simulink model "uplink_4c1r"  (Simulink 8.7)
settings: Solver=VariableStepDiscrete  StartTime=0.0  StopTime=DDC_Lineup_param.endTime  RelTol=1e-3
PreLoadFcn:
  | % Run the setup script when the model is opened
  | setup_uplink_4c1r;
InitFcn:
  | % Run the setup script again just before the
  | % model is run, so that any updates made
  | % after opening are applied.
  | setup_uplink_4c1r;
  | %% DSPBuilder Start
  | alt_dspbuilder_update_model(bdroot)
  | %% DSPBuilder End
undefined symbols (not defined in the file or in its folder): AdvDSPBChannelOutDisplay, carrier_separation, DDC_Lineup_param, dpoly, dspba_ChannelInVis, dspba_ChannelOutVis, dspba_internal_get_channel_ports, dspba_internal_get_demux_ports, evalAionMaskParam, latency, Power_Meter, primtype, Subsystem, uplink_4c1r_carrier_seperation_4c, uplink_4c1r_pd_accu_reg_block, uplink_4c1r_power_meter_1carrier, value
undefined symbols (not defined in the file): power_meter_param
libraries: DSPBAPrim x119, DSPBABase x26, uplink_4c1r_pipereg_lib x22, DSPBAModelBus x9, DSPBAFilters x5, uplink_4c1r_register x5, uplink_4c1r_accumulator x5, uplink_4c1r_peak_detector x5, uplink_4c1r_iq_square x4, DSPBAControl x2, DSPBAWaveformSynth x2, DSPBAUtilities x1
(part 2 of 3)

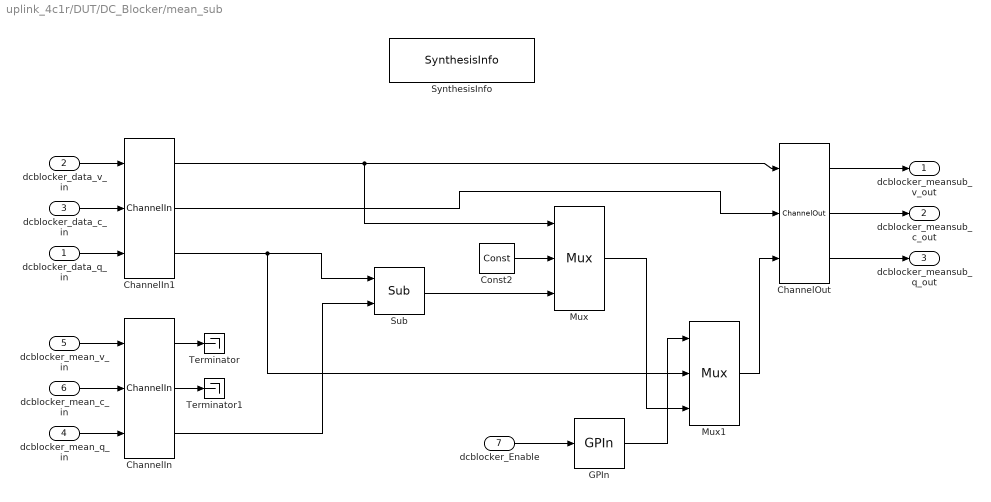
== system uplink_4c1r/DUT/DC_Blocker/mean_sub ==
  dcblocker_data_q_in : Inport
  dcblocker_data_v_in : Inport  Port=2
  dcblocker_data_c_in : Inport  Port=3
  dcblocker_mean_q_in : Inport  Port=4
  dcblocker_mean_v_in : Inport  Port=5
  dcblocker_mean_c_in : Inport  Port=6
  dcblocker_Enable : Inport  Port=7
  ChannelIn : DSPBAPrim/ChannelIn  primtype=channelin  nInputs=dspba_internal_get_channel_ports(gcb)  nOutputs=dspba_internal_get_channel_ports(gcb)  omode=Inherit via internal rule  otype=sfix(16)  scale=2^-15  rndmethod=Unbiased  factor=1  satmethod=Symmetric  shift_vec=[0 1 2 -1]  value=1  inPortNames=['v'; 'c'; '0'; '1'; '2'; '3'; '4'; '5'; '6'; '7'; '8'; '9'; 'A'; 'B'; 'D'; 'E'; 'F'; 'G'; 'H'; 'I'; 'J'; 'K'; 'L'; 'M'; 'N'; 'O'; 'P'; 'Q'; 'R'; 'S'; 'T'; 'U'; 'W'; 'X'; 'Y'; 'Z']  outPortNames=['v'; 'c'; '0'; '1'; '2'; '3'; '4'; '5'; '6'; '7'; '8'; '9'; 'A'; 'B'; 'D'; 'E'; 'F'; 'G'; 'H'; 'I'; 'J'; 'K'; 'L'; 'M'; 'N'; 'O'; 'P'; 'Q'; 'R'; 'S'; 'T'; 'U'; 'W'; 'X'; 'Y'; 'Z']  dspbaimage=dspba_prim.jpg  text=fprintf('In');  style=Optimised  dataSignals=1  foldingEnabled=off  channels=1  sampleRate=200  packetBeginPresent=off  packetBeginEnabled=off  visibilities=dspba_ChannelInVis(gcb)  latencyCorrection=0  version=20141013
  ChannelIn1 : DSPBAPrim/ChannelIn  primtype=channelin  nInputs=dspba_internal_get_channel_ports(gcb)  nOutputs=dspba_internal_get_channel_ports(gcb)  omode=Inherit via internal rule  otype=sfix(16)  scale=2^-15  rndmethod=Unbiased  factor=1  satmethod=Symmetric  shift_vec=[0 1 2 -1]  value=1  inPortNames=['v'; 'c'; '0'; '1'; '2'; '3'; '4'; '5'; '6'; '7'; '8'; '9'; 'A'; 'B'; 'D'; 'E'; 'F'; 'G'; 'H'; 'I'; 'J'; 'K'; 'L'; 'M'; 'N'; 'O'; 'P'; 'Q'; 'R'; 'S'; 'T'; 'U'; 'W'; 'X'; 'Y'; 'Z']  outPortNames=['v'; 'c'; '0'; '1'; '2'; '3'; '4'; '5'; '6'; '7'; '8'; '9'; 'A'; 'B'; 'D'; 'E'; 'F'; 'G'; 'H'; 'I'; 'J'; 'K'; 'L'; 'M'; 'N'; 'O'; 'P'; 'Q'; 'R'; 'S'; 'T'; 'U'; 'W'; 'X'; 'Y'; 'Z']  dspbaimage=dspba_prim.jpg  text=fprintf('In');  style=Optimised  dataSignals=1  foldingEnabled=off  channels=1  sampleRate=200  packetBeginPresent=off  packetBeginEnabled=off  visibilities=dspba_ChannelInVis(gcb)  latencyCorrection=0  version=20141013
  ChannelOut : DSPBAPrim/ChannelOut  primtype=channelout  nInputs=dspba_internal_get_channel_ports(gcb)  nOutputs=dspba_internal_get_channel_ports(gcb)  omode=Inherit via internal rule  otype=sfix(16)  scale=2^-15  rndmethod=Unbiased  factor=1  satmethod=Symmetric  shift_vec=[0 1 2 -1]  value=1  inPortNames=['v'; 'c'; '0'; '1'; '2'; '3'; '4'; '5'; '6'; '7'; '8'; '9'; 'A'; 'B'; 'D'; 'E'; 'F'; 'G'; 'H'; 'I'; 'J'; 'K'; 'L'; 'M'; 'N'; 'O'; 'P'; 'Q'; 'R'; 'S'; 'T'; 'U'; 'W'; 'X'; 'Y'; 'Z']  outPortNames=['v'; 'c'; '0'; '1'; '2'; '3'; '4'; '5'; '6'; '7'; '8'; '9'; 'A'; 'B'; 'D'; 'E'; 'F'; 'G'; 'H'; 'I'; 'J'; 'K'; 'L'; 'M'; 'N'; 'O'; 'P'; 'Q'; 'R'; 'S'; 'T'; 'U'; 'W'; 'X'; 'Y'; 'Z']  dspbaimage=dspba_prim.jpg  text=fprintf('Out%s', AdvDSPBChannelOutDisplay(latency));  style=Optimised  dataSignals=1  foldingEnabled=off  channels=1  sampleRate=200  packetBeginPresent=off  packetBeginEnabled=off  visibilities=dspba_ChannelOutVis(gcb)  latency=21  latencyCorrection=0  version=20141013
  Const2 : DSPBAPrim/Const  primtype=const  nInputs=0  nOutputs=1  omode=Specify via dialog  otype=sfix(16)  scale=2^-15  rndmethod=Unbiased  factor=1  satmethod=Symmetric  shift_vec=[0 1 2 -1]  value=0  inPortNames=['+'; '+';]  outPortNames=[' ']  dspbaimage=dspba_prim.jpg  text=fprintf('%s', num2str(value));  style=Optimised  visibilities=8 + 1024  floatPrecision=float32_m23  version=20120820
  GPIn : DSPBAPrim/GPIn  primtype=gpin  nInputs=evalAionMaskParam(gcb,'value',1)  nOutputs=evalAionMaskParam(gcb,'value',1)  omode=Inherit via internal rule  otype=sfix(16)  scale=2^-15  rndmethod=Unbiased  factor=1  satmethod=Symmetric  shift_vec=[0 1 2 -1]  value=1  inPortNames=[' ' ' ' ' ' ' ' ' ' ' ' ' ' ' ' ' ' ' ' ' ' ' ' ' ' ' ' ' ' ' ' ' ' ' ' ' ' ' ' ' ' ' ' ' ' ' ' ' ' ' ' ' ' ' ' ' ' ' ' ' ' ' ' ' ' ' ' ' ']'  outPortNames=[' ' ' ' ' ' ' ' ' ' ' ' ' ' ' ' ' ' ' ' ' ' ' ' ' ' ' ' ' ' ' ' ' ' ' ' ' ' ' ' ' ' ' ' ' ' ' ' ' ' ' ' ' ' ' ' ' ' ' ' ' ' ' ' ' ' ' ' ' ']'  dspbaimage=dspba_prim.jpg  text=fprintf('GPIn');  style=Optimised  visibilities=1024  latencyCorrection=0  version=20090407
  Mux : DSPBAPrim/Mux  primtype=mux  nInputs=evalAionMaskParam(gcb,'value',1)+1  nOutputs=1  omode=Inherit via internal rule  otype=sfix(16)  scale=2^-15  rndmethod=Unbiased  factor=1  satmethod=Symmetric  shift_vec=[0 1 2 -1]  value=2  inPortNames=['s'; 'd0'; 'd1'; 'd2'; 'd3'; 'd4'; 'd5'; 'd6'; 'd7'; 'd8'; 'd9';]  outPortNames=[' ']  dspbaimage=dspba_prim.jpg  text=fprintf('%s', primtype);  style=Optimised  visibilities=1032  version=20131025
  Mux1 : DSPBAPrim/Mux  primtype=mux  nInputs=evalAionMaskParam(gcb,'value',1)+1  nOutputs=1  omode=Inherit via internal rule  otype=sfix(16)  scale=2^-15  rndmethod=Unbiased  factor=1  satmethod=Symmetric  shift_vec=[0 1 2 -1]  value=2  inPortNames=['s'; 'd0'; 'd1'; 'd2'; 'd3'; 'd4'; 'd5'; 'd6'; 'd7'; 'd8'; 'd9';]  outPortNames=[' ']  dspbaimage=dspba_prim.jpg  text=fprintf('%s', primtype);  style=Optimised  visibilities=1032  version=20131025
  Sub : DSPBAPrim/Sub  primtype=sub  nInputs=2  nOutputs=1  omode=Inherit via internal rule  otype=sfix(16)  scale=2^-15  rndmethod=Unbiased  factor=1  satmethod=Symmetric  shift_vec=[0 1 2 -1]  value=0  inPortNames=['+'; '-';]  outPortNames=[' ']  dspbaimage=dspba_prim.jpg  text=fprintf('-');  style=Optimised  visibilities=8+2^17+2^18  floatRounding=correct  advOptions=[]  version=20130115
  SynthesisInfo : DSPBAPrim/SynthesisInfo  primtype=synthinfo  nInputs=0  nOutputs=0  omode=Inherit via internal rule  otype=sfix(16)  scale=2^-15  rndmethod=Truncate  factor=1  satmethod=Symmetric  shift_vec=[0 1 2 -1]  value=99  inPortNames=[' '; ' ';]  outPortNames=[' ']  dspbaimage=dspba_prim_ctrl.jpg  text=fprintf('Style=%s', style);  style=Scheduled  visibilities=2^15+2^17+2^18+2^19  constraintInUse=on  constraintRelation=>  constraintLimit=20  bitAccurate=off  version=20150220
  Terminator : Terminator
  Terminator1 : Terminator
  dcblocker_meansub_v_out : Outport
  dcblocker_meansub_c_out : Outport  Port=2
  dcblocker_meansub_q_out : Outport  Port=3
  wires:
  dcblocker_mean_c_in/1 -> ChannelIn/2
  dcblocker_mean_v_in/1 -> ChannelIn/1
  dcblocker_mean_q_in/1 -> ChannelIn/3
  ChannelOut/1 -> dcblocker_meansub_v_out/1
  ChannelOut/3 -> dcblocker_meansub_q_out/1
  ChannelOut/2 -> dcblocker_meansub_c_out/1
  dcblocker_data_c_in/1 -> ChannelIn1/2
  dcblocker_data_v_in/1 -> ChannelIn1/1
  dcblocker_data_q_in/1 -> ChannelIn1/3
  ChannelIn1/3 -> Mux1/2, Sub/1
  ChannelIn/3 -> Sub/2
  ChannelIn/1 -> Terminator/1
  ChannelIn/2 -> Terminator1/1
  Sub/1 -> Mux/3
  Const2/1 -> Mux/2
  ChannelIn1/1 -> ChannelOut/1, Mux/1
  ChannelIn1/2 -> ChannelOut/2
  Mux/1 -> Mux1/3
  Mux1/1 -> ChannelOut/3
  dcblocker_Enable/1 -> GPIn/1
  GPIn/1 -> Mux1/1

== system uplink_4c1r/DUT/DDC/Chan_Filter ==
  In_a : Inport
  In_V : Inport  Port=2
  In_C : Inport  Port=3
  Const2 : DSPBAPrim/Const  primtype=const  nInputs=0  nOutputs=1  omode=Inherit via internal rule  otype=sfix(16)  scale=2^-15  rndmethod=Unbiased  factor=1  satmethod=Symmetric  shift_vec=[0 1 2 -1]  value=0  inPortNames=['+'; '+';]  outPortNames=[' ']  dspbaimage=dspba_prim.jpg  text=fprintf('%s', num2str(value));  style=Optimised  visibilities=8 + 1024  floatPrecision=float32_m23  version=20120820
  Terminator2 : Terminator
  chan_filter1_Scale1 : DSPBABase/Scale  otype=sfix(DDC_Lineup_param.output_word_length)  scale=2^-DDC_Lineup_param.output_fraction_length  rndmethod=Truncate  factor=1  satmethod=Symmetric  shift_vec=0  latency=4  wideSimulation=off  version=20130807
  chan_filter6 : DSPBAFilters/SingleRateFIR  nInputRate=DDC_Lineup_param.CH_filter.SampleRate  nchan=DDC_Lineup_param.CH_filter.ChanCount  symmetry=Symmetrical  coef=DDC_Lineup_param.chan_filter.coeffs(1,:)  addr=DDC_Lineup_param.CH_filter.base_addr1  rwmode=Read/Write  nband=Use All Taps  latency=22  exposebus=off  version=20090407  recon=off  MM=[0,1,2,3,4,5,6,7,8,9,10,11,12,13,14,15,16,17,18,19]
  data_out : Outport
  valid_out : Outport  Port=2
  chan_out : Outport  Port=3
  wires:
  chan_filter6/2 -> chan_filter1_Scale1/2
  chan_filter6/3 -> chan_filter1_Scale1/3
  chan_filter1_Scale1/2 -> valid_out/1
  Const2/1 -> chan_filter1_Scale1/4
  chan_filter1_Scale1/1 -> data_out/1
  chan_filter1_Scale1/4 -> Terminator2/1
  chan_filter1_Scale1/3 -> chan_out/1
  chan_filter6/1 -> chan_filter1_Scale1/1
  In_C/1 -> chan_filter6/3
  In_V/1 -> chan_filter6/2
  In_a/1 -> chan_filter6/1

== system uplink_4c1r/DUT/DDC/HB4 ==
  In_Data : Inport
  In_Valid : Inport  Port=2
  In_Chan : Inport  Port=3
  Const9 : DSPBAPrim/Const  primtype=const  nInputs=0  nOutputs=1  omode=Inherit via internal rule  otype=sfix(16)  scale=2^-15  rndmethod=Unbiased  factor=1  satmethod=Symmetric  shift_vec=[0 1 2 -1]  value=0  inPortNames=['+'; '+';]  outPortNames=[' ']  dspbaimage=dspba_prim.jpg  text=fprintf('%s', num2str(value));  style=Optimised  visibilities=8 + 1024  floatPrecision=float32_m23  version=20120820
  HB_4 : DSPBAFilters/DecimatingFIR  nInputRate=DDC_Lineup_param.HB_filter4.SampleRate  decim=DDC_Lineup_param.HB_filter4.Decimation  nchan=DDC_Lineup_param.HB_filter4.ChanCount  symmetry=Symmetrical  coef=DDC_Lineup_param.HB_filt4.coeffs(1,:)  addr=DDC_Lineup_param.HB_filter4.base_addr1  rwmode=Read/Write  nband=Half Band  exposebus=off  latency=22  version=20090407  recon=off  MM=[0,1,2,3,4,5,6,7,8,9,10,11,12,13,14,15]
  HB_4_Scale : DSPBABase/Scale  otype=sfix(DDC_Lineup_param.output_word_length)  scale=2^-DDC_Lineup_param.output_fraction_length  rndmethod=Truncate  factor=1  satmethod=Symmetric  shift_vec=0  latency=4  wideSimulation=off  version=20130807
  Terminator10 : Terminator
  Terminator4 : Terminator
  Out_Data : Outport
  Out_Valid : Outport  Port=2
  Out_Chan : Outport  Port=3
  wires:
  HB_4/3 -> HB_4_Scale/3
  HB_4/1 -> HB_4_Scale/1
  HB_4/2 -> HB_4_Scale/2
  Const9/1 -> HB_4_Scale/4
  HB_4_Scale/4 -> Terminator4/1
  In_Valid/1 -> HB_4/2
  In_Chan/1 -> HB_4/3
  In_Data/1 -> HB_4/1
  HB_4_Scale/1 -> Out_Data/1
  HB_4_Scale/3 -> Out_Chan/1
  HB_4_Scale/2 -> Out_Valid/1

== system uplink_4c1r/DUT/DDC/HB5 ==
  In_Data : Inport
  In_Valid : Inport  Port=2
  In_Chan : Inport  Port=3
  Const10 : DSPBAPrim/Const  primtype=const  nInputs=0  nOutputs=1  omode=Inherit via internal rule  otype=sfix(16)  scale=2^-15  rndmethod=Unbiased  factor=1  satmethod=Symmetric  shift_vec=[0 1 2 -1]  value=0  inPortNames=['+'; '+';]  outPortNames=[' ']  dspbaimage=dspba_prim.jpg  text=fprintf('%s', num2str(value));  style=Optimised  visibilities=8 + 1024  floatPrecision=float32_m23  version=20120820
  HB5_Scale : DSPBABase/Scale  otype=sfix(DDC_Lineup_param.output_word_length)  scale=2^-DDC_Lineup_param.output_fraction_length  rndmethod=Truncate  factor=1  satmethod=Symmetric  shift_vec=0  latency=4  wideSimulation=off  version=20130807
  HB_5_1 : DSPBAFilters/DecimatingFIR  nInputRate=DDC_Lineup_param.HB_filter5.SampleRate  decim=DDC_Lineup_param.HB_filter5.Decimation  nchan=DDC_Lineup_param.HB_filter5.ChanCount  symmetry=Symmetrical  coef=DDC_Lineup_param.HB_filt5.coeffs(1,:)  addr=DDC_Lineup_param.HB_filter5.base_addr1  rwmode=Read/Write  nband=Half Band  exposebus=off  latency=21  version=20090407  recon=off  MM=[0,1,2,3,4,5,6,7,8,9,10,11,12,13,14,15]
  Terminator11 : Terminator
  Out_Data : Outport
  Out_Valid : Outport  Port=2
  Out_Chan : Outport  Port=3
  wires:
  HB5_Scale/4 -> Terminator11/1
  HB_5_1/3 -> HB5_Scale/3
  HB_5_1/2 -> HB5_Scale/2
  Const10/1 -> HB5_Scale/4
  HB_5_1/1 -> HB5_Scale/1
  HB5_Scale/2 -> Out_Valid/1
  HB5_Scale/3 -> Out_Chan/1
  HB5_Scale/1 -> Out_Data/1
  In_Valid/1 -> HB_5_1/2
  In_Chan/1 -> HB_5_1/3
  In_Data/1 -> HB_5_1/1

== system uplink_4c1r/DUT/DDC/HB6 ==
  In_Data : Inport
  In_Valid : Inport  Port=2
  In_Chan : Inport  Port=3
  Const19 : DSPBAPrim/Const  primtype=const  nInputs=0  nOutputs=1  omode=Specify via dialog  otype=ufix(1)  scale=2^-0  rndmethod=Unbiased  factor=1  satmethod=Symmetric  shift_vec=[0 1 2 -1]  value=0  inPortNames=['+'; '+';]  outPortNames=[' ']  dspbaimage=dspba_prim.jpg  text=fprintf('%s', num2str(value));  style=Optimised  visibilities=8 + 1024  floatPrecision=float32_m23  version=20120820
  HB_6 : DSPBAFilters/DecimatingFIR  nInputRate=DDC_Lineup_param.HB_filter6.SampleRate  decim=DDC_Lineup_param.HB_filter6.Decimation  nchan=DDC_Lineup_param.HB_filter6.ChanCount  symmetry=Symmetrical  coef=DDC_Lineup_param.HB_filt6.coeffs(1,:)  addr=DDC_Lineup_param.HB_filter6.base_addr1  rwmode=Read/Write  nband=Half Band  exposebus=off  latency=14  version=20090407  recon=off  MM=[0,1,2,3,4,5,6,7,8,9,10,11,12,13,14,15]
  HB_6_Scale : DSPBABase/Scale  otype=sfix(DDC_Lineup_param.output_word_length)  scale=2^-DDC_Lineup_param.output_fraction_length  rndmethod=Truncate  factor=1  satmethod=Symmetric  shift_vec=0  latency=4  wideSimulation=off  version=20130807
  Terminator12 : Terminator
  Out_Data1 : Outport
  Valid : Outport  Port=2
  Chan : Outport  Port=3
  wires:
  HB_6_Scale/1 -> Out_Data1/1
  Const19/1 -> HB_6_Scale/4
  HB_6_Scale/4 -> Terminator12/1
  HB_6/3 -> HB_6_Scale/3
  HB_6_Scale/3 -> Chan/1
  HB_6/1 -> HB_6_Scale/1
  HB_6/2 -> HB_6_Scale/2
  HB_6_Scale/2 -> Valid/1
  In_Valid/1 -> HB_6/2
  In_Chan/1 -> HB_6/3
  In_Data/1 -> HB_6/1

== system uplink_4c1r/DUT/DDC/HB7 ==
  In_Data : Inport
  In_Valid : Inport  Port=2
  In_Chan : Inport  Port=3
  Const19 : DSPBAPrim/Const  primtype=const  nInputs=0  nOutputs=1  omode=Specify via dialog  otype=ufix(1)  scale=2^-0  rndmethod=Unbiased  factor=1  satmethod=Symmetric  shift_vec=[0 1 2 -1]  value=0  inPortNames=['+'; '+';]  outPortNames=[' ']  dspbaimage=dspba_prim.jpg  text=fprintf('%s', num2str(value));  style=Optimised  visibilities=8 + 1024  floatPrecision=float32_m23  version=20120820
  HB_7 : DSPBAFilters/DecimatingFIR  nInputRate=DDC_Lineup_param.HB_filter7.SampleRate  decim=DDC_Lineup_param.HB_filter7.Decimation  nchan=DDC_Lineup_param.HB_filter7.ChanCount  symmetry=Symmetrical  coef=DDC_Lineup_param.HB_filt7.coeffs(1,:)  addr=DDC_Lineup_param.HB_filter7.base_addr  rwmode=Read/Write  nband=Half Band  exposebus=off  latency=17  version=20090407  recon=off  MM=[0,1,2,3,4,5,6,7,8,9,10,11,12,13,14,15]
  HB_7_Scale : DSPBABase/Scale  otype=sfix(DDC_Lineup_param.output_word_length)  scale=2^-DDC_Lineup_param.output_fraction_length  rndmethod=Truncate  factor=1  satmethod=Symmetric  shift_vec=0  latency=4  wideSimulation=off  version=20130807
  Terminator12 : Terminator
  Out_Data1 : Outport
  Valid : Outport  Port=2
  Chan : Outport  Port=3
  wires:
  In_Data/1 -> HB_7/1
  In_Chan/1 -> HB_7/3
  In_Valid/1 -> HB_7/2
  HB_7_Scale/2 -> Valid/1
  HB_7/2 -> HB_7_Scale/2
  HB_7/1 -> HB_7_Scale/1
  HB_7_Scale/3 -> Chan/1
  HB_7/3 -> HB_7_Scale/3
  HB_7_Scale/4 -> Terminator12/1
  Const19/1 -> HB_7_Scale/4
  HB_7_Scale/1 -> Out_Data1/1

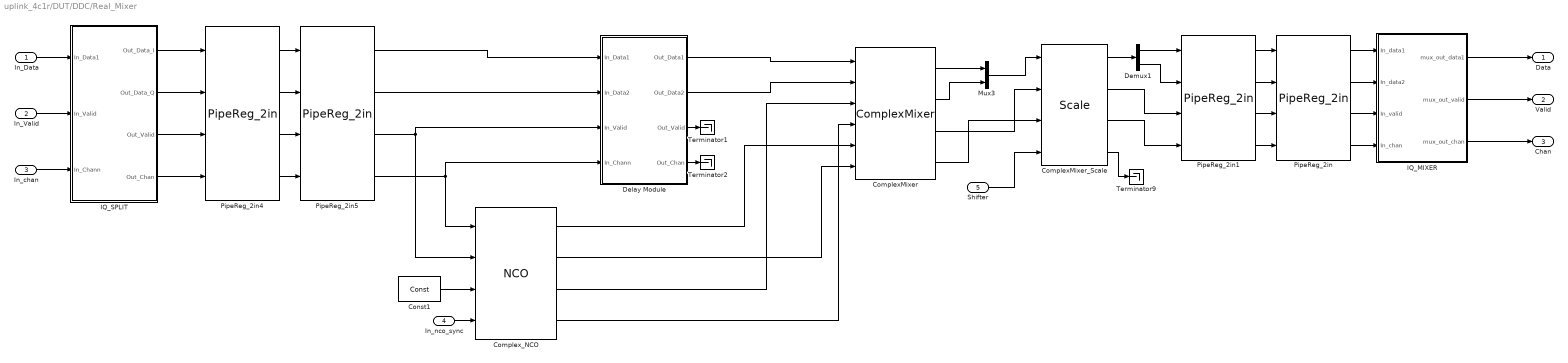
== system uplink_4c1r/DUT/DDC/Real_Mixer ==
  In_Data : Inport
  "In_Valid " : Inport  Port=2
  "In_chan " : Inport  Port=3
  In_nco_sync : Inport  Port=4
  Shifter : Inport  Port=5
  ComplexMixer : DSPBAWaveformSynth/ComplexMixer  nInputRate=DDC_Lineup_param.RM.SampleRate  nchan=DDC_Lineup_param.RM.No_Of_complex_chan  nfreq=DDC_Lineup_param.RM.No_Of_complex_Freq  latency=4  version=20090407
  ComplexMixer_Scale : DSPBABase/Scale  otype=sfix(DDC_Lineup_param.output_word_length)  scale=2^-DDC_Lineup_param.output_fraction_length  rndmethod=Truncate  factor=[1 1 1 1]  satmethod=Symmetric  shift_vec=[0 1 2 3]  latency=7  wideSimulation=off  version=20130807
  Complex_NCO : DSPBAWaveformSynth/NCO  outputRate=DDC_Lineup_param.Complex_NCO_A1.SampleRate  otype=sfix(DDC_Lineup_param.Complex_NCO_A1.Data_type)  scale=2^-DDC_Lineup_param.Complex_NCO_A1.scaling_value  expSFDR=96.32  accumBitWidth=DDC_Lineup_param.Complex_NCO_A1.Acumulater_bit_wid  accumPrecision=+/- 3.6621  phaseIncrAndInv=DDC_Lineup_param.Complex_NCO_A1.Freq_word  phaseIncrInMHz="[0  0  0  0]"  phaseIncrAndInvMap=DDC_Lineup_param.Complex_NCO_A1.base_addr  rwmode=Read/Write  exposebus=off  outWidth=1  tableSize=8  latency=18  version=20090407
  Const1 : DSPBAPrim/Const  primtype=const  nInputs=0  nOutputs=1  omode=Specify via dialog  otype=ufix(24)  scale=2^-0  rndmethod=Unbiased  factor=1  satmethod=Symmetric  shift_vec=[0 1 2 -1]  value=0  inPortNames=['+'; '+';]  outPortNames=[' ']  dspbaimage=dspba_prim.jpg  text=fprintf('%s', num2str(value));  style=Optimised  visibilities=8 + 1024  floatPrecision=float32_m23  version=20120820
  Delay Module : Subsystem
  Demux1 : Demux  Outputs=2
  IQ_MIXER : Subsystem
  IQ_SPLIT : Subsystem
  Mux3 : Mux  Inputs=2
  PipeReg_2in : uplink_4c1r_pipereg_lib/PipeReg_2in  NPipe=2  Clock_Margin=100
      link override ChannelOut: value=2  packetBeginEnabled=off  latency=2
  PipeReg_2in1 : uplink_4c1r_pipereg_lib/PipeReg_2in  NPipe=2  Clock_Margin=100
      link override ChannelOut: value=2  packetBeginEnabled=off  latency=2
  PipeReg_2in4 : uplink_4c1r_pipereg_lib/PipeReg_2in  NPipe=1  Clock_Margin=100
      link override ChannelOut: value=2  packetBeginEnabled=off  latency=1
  PipeReg_2in5 : uplink_4c1r_pipereg_lib/PipeReg_2in  NPipe=1  Clock_Margin=100
      link override ChannelOut: value=2  packetBeginEnabled=off  latency=1
  Terminator1 : Terminator
  Terminator2 : Terminator
  Terminator9 : Terminator
  Data : Outport
  Valid : Outport  Port=2
  Chan : Outport  Port=3
  wires:
  ComplexMixer_Scale/4 -> Terminator9/1
  Mux3/1 -> ComplexMixer_Scale/1
  ComplexMixer/4 -> ComplexMixer_Scale/3
  ComplexMixer/3 -> ComplexMixer_Scale/2
  Shifter/1 -> ComplexMixer_Scale/4
  ComplexMixer/1 -> Mux3/1
  ComplexMixer/2 -> Mux3/2
  ComplexMixer_Scale/1 -> Demux1/1
  IQ_MIXER/2(mux_out_valid) -> Valid/1
  IQ_MIXER/3(mux_out_chan) -> Chan/1
  IQ_MIXER/1(mux_out_data1) -> Data/1
  "In_chan "/1 -> IQ_SPLIT/3(In_Chann)
  In_nco_sync/1 -> Complex_NCO/4
  Const1/1 -> Complex_NCO/3
  "In_Valid "/1 -> IQ_SPLIT/2(In_Valid)
  In_Data/1 -> IQ_SPLIT/1(In_Data1)
  PipeReg_2in5/3 -> Complex_NCO/2, Delay Module/3(In_Valid)
  PipeReg_2in5/4 -> Complex_NCO/1, Delay Module/4(In_Chann)
  PipeReg_2in/1 -> IQ_MIXER/1(In_data1)
  PipeReg_2in/2 -> IQ_MIXER/2(In_data2)
  PipeReg_2in/3 -> IQ_MIXER/3(In_valid)
  PipeReg_2in/4 -> IQ_MIXER/4(In_chan)
  PipeReg_2in1/1 -> PipeReg_2in/1
  PipeReg_2in1/2 -> PipeReg_2in/2
  PipeReg_2in1/3 -> PipeReg_2in/3
  PipeReg_2in1/4 -> PipeReg_2in/4
  Demux1/1 -> PipeReg_2in1/1
  Demux1/2 -> PipeReg_2in1/2
  ComplexMixer_Scale/2 -> PipeReg_2in1/3
  ComplexMixer_Scale/3 -> PipeReg_2in1/4
  Complex_NCO/2 -> ComplexMixer/6
  Complex_NCO/3 -> ComplexMixer/3
  Complex_NCO/4 -> ComplexMixer/4
  Complex_NCO/1 -> ComplexMixer/5
  IQ_SPLIT/1(Out_Data_I) -> PipeReg_2in4/1
  IQ_SPLIT/4(Out_Chan) -> PipeReg_2in4/4
  PipeReg_2in4/1 -> PipeReg_2in5/1
  PipeReg_2in4/2 -> PipeReg_2in5/2
  PipeReg_2in4/3 -> PipeReg_2in5/3
  PipeReg_2in4/4 -> PipeReg_2in5/4
  IQ_SPLIT/2(Out_Data_Q) -> PipeReg_2in4/2
  IQ_SPLIT/3(Out_Valid) -> PipeReg_2in4/3
  Delay Module/1(Out_Data1) -> ComplexMixer/1
  Delay Module/2(Out_Data2) -> ComplexMixer/2
  PipeReg_2in5/1 -> Delay Module/1(In_Data1)
  PipeReg_2in5/2 -> Delay Module/2(In_Data2)
  Delay Module/3(Out_Valid) -> Terminator1/1
  Delay Module/4(Out_Chan) -> Terminator2/1

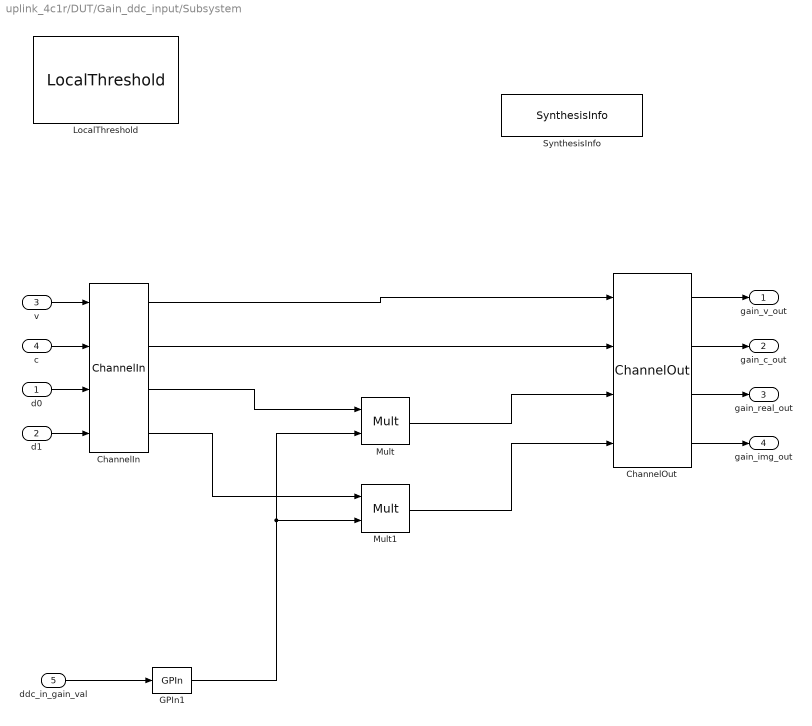
== system uplink_4c1r/DUT/Gain_ddc_input/Subsystem ==
  d0 : Inport
  d1 : Inport  Port=2
  v : Inport  Port=3
  c : Inport  Port=4
  ddc_in_gain_val : Inport  Port=5
  ChannelIn : DSPBAPrim/ChannelIn  primtype=channelin  nInputs=dspba_internal_get_channel_ports(gcb)  nOutputs=dspba_internal_get_channel_ports(gcb)  omode=Inherit via internal rule  otype=sfix(16)  scale=2^-15  rndmethod=Unbiased  factor=1  satmethod=Symmetric  shift_vec=[0 1 2 -1]  value=2  inPortNames=['v'; 'c'; '0'; '1'; '2'; '3'; '4'; '5'; '6'; '7'; '8'; '9'; 'A'; 'B'; 'D'; 'E'; 'F'; 'G'; 'H'; 'I'; 'J'; 'K'; 'L'; 'M'; 'N'; 'O'; 'P'; 'Q'; 'R'; 'S'; 'T'; 'U'; 'W'; 'X'; 'Y'; 'Z']  outPortNames=['v'; 'c'; '0'; '1'; '2'; '3'; '4'; '5'; '6'; '7'; '8'; '9'; 'A'; 'B'; 'D'; 'E'; 'F'; 'G'; 'H'; 'I'; 'J'; 'K'; 'L'; 'M'; 'N'; 'O'; 'P'; 'Q'; 'R'; 'S'; 'T'; 'U'; 'W'; 'X'; 'Y'; 'Z']  dspbaimage=dspba_prim.jpg  text=fprintf('In');  style=Optimised  dataSignals=2  foldingEnabled=off  channels=1  sampleRate=200  packetBeginPresent=off  packetBeginEnabled=off  visibilities=dspba_ChannelInVis(gcb)  latencyCorrection=0  version=20141013
  ChannelOut : DSPBAPrim/ChannelOut  primtype=channelout  nInputs=dspba_internal_get_channel_ports(gcb)  nOutputs=dspba_internal_get_channel_ports(gcb)  omode=Inherit via internal rule  otype=sfix(16)  scale=2^-15  rndmethod=Unbiased  factor=1  satmethod=Symmetric  shift_vec=[0 1 2 -1]  value=2  inPortNames=['v'; 'c'; '0'; '1'; '2'; '3'; '4'; '5'; '6'; '7'; '8'; '9'; 'A'; 'B'; 'D'; 'E'; 'F'; 'G'; 'H'; 'I'; 'J'; 'K'; 'L'; 'M'; 'N'; 'O'; 'P'; 'Q'; 'R'; 'S'; 'T'; 'U'; 'W'; 'X'; 'Y'; 'Z']  outPortNames=['v'; 'c'; '0'; '1'; '2'; '3'; '4'; '5'; '6'; '7'; '8'; '9'; 'A'; 'B'; 'D'; 'E'; 'F'; 'G'; 'H'; 'I'; 'J'; 'K'; 'L'; 'M'; 'N'; 'O'; 'P'; 'Q'; 'R'; 'S'; 'T'; 'U'; 'W'; 'X'; 'Y'; 'Z']  dspbaimage=dspba_prim.jpg  text=fprintf('Out%s', AdvDSPBChannelOutDisplay(latency));  style=Optimised  dataSignals=2  foldingEnabled=off  channels=1  sampleRate=200  packetBeginPresent=off  packetBeginEnabled=off  visibilities=dspba_ChannelOutVis(gcb)  latency=21  latencyCorrection=0  version=20141013
  GPIn1 : DSPBAPrim/GPIn  primtype=gpin  nInputs=evalAionMaskParam(gcb,'value',1)  nOutputs=evalAionMaskParam(gcb,'value',1)  omode=Inherit via internal rule  otype=sfix(16)  scale=2^-15  rndmethod=Unbiased  factor=1  satmethod=Symmetric  shift_vec=[0 1 2 -1]  value=1  inPortNames=[' ' ' ' ' ' ' ' ' ' ' ' ' ' ' ' ' ' ' ' ' ' ' ' ' ' ' ' ' ' ' ' ' ' ' ' ' ' ' ' ' ' ' ' ' ' ' ' ' ' ' ' ' ' ' ' ' ' ' ' ' ' ' ' ' ' ' ' ' ']'  outPortNames=[' ' ' ' ' ' ' ' ' ' ' ' ' ' ' ' ' ' ' ' ' ' ' ' ' ' ' ' ' ' ' ' ' ' ' ' ' ' ' ' ' ' ' ' ' ' ' ' ' ' ' ' ' ' ' ' ' ' ' ' ' ' ' ' ' ' ' ' ' ']'  dspbaimage=dspba_prim.jpg  text=fprintf('GPIn');  style=Optimised  visibilities=1024  latencyCorrection=0  version=20090407
  LocalThreshold : DSPBABase/LocalThreshold  margin=DDC_Lineup_param.ClockMargin  delayRegOrRAMThresholdBits=-1  MediumDualMemThresholdBits=-1  LargeDualMemThresholdBits=-1  hardMultiplierThresholdLuts=-1  complexMultKaratsuba=off  version=0
  Mult : DSPBAPrim/Mult  primtype=mult  nInputs=2  nOutputs=1  omode=Inherit via internal rule  otype=sfix(16)  scale=2^-15  rndmethod=Unbiased  factor=1  satmethod=Symmetric  shift_vec=[0 1 2 -1]  value=0  inPortNames=[' '; ' ';]  outPortNames=[' ']  dspbaimage=dspba_prim.jpg  text=fprintf('X');  style=Optimised  visibilities=8+2^18+2^19  floatPrecision=float32_m23  floatRounding=correct  advOptions=[]  version=20130115
  Mult1 : DSPBAPrim/Mult  primtype=mult  nInputs=2  nOutputs=1  omode=Inherit via internal rule  otype=sfix(16)  scale=2^-15  rndmethod=Unbiased  factor=1  satmethod=Symmetric  shift_vec=[0 1 2 -1]  value=0  inPortNames=[' '; ' ';]  outPortNames=[' ']  dspbaimage=dspba_prim.jpg  text=fprintf('X');  style=Optimised  visibilities=8+2^18+2^19  floatPrecision=float32_m23  floatRounding=correct  advOptions=[]  version=20130115
  SynthesisInfo : DSPBAPrim/SynthesisInfo  primtype=synthinfo  nInputs=0  nOutputs=0  omode=Inherit via internal rule  otype=sfix(16)  scale=2^-15  rndmethod=Truncate  factor=1  satmethod=Symmetric  shift_vec=[0 1 2 -1]  value=99  inPortNames=[' '; ' ';]  outPortNames=[' ']  dspbaimage=dspba_prim_ctrl.jpg  text=fprintf('Style=%s', style);  style=Scheduled  visibilities=2^15+2^17+2^18+2^19  constraintInUse=on  constraintRelation=>  constraintLimit=20  bitAccurate=off  version=20150220
  gain_v_out : Outport
  gain_c_out : Outport  Port=2
  gain_real_out : Outport  Port=3
  gain_img_out : Outport  Port=4
  wires:
  GPIn1/1 -> Mult1/2, Mult/2
  ddc_in_gain_val/1 -> GPIn1/1
  v/1 -> ChannelIn/1
  c/1 -> ChannelIn/2
  d0/1 -> ChannelIn/3
  d1/1 -> ChannelIn/4
  ChannelIn/3 -> Mult/1
  ChannelIn/4 -> Mult1/1
  ChannelOut/1 -> gain_v_out/1
  ChannelOut/2 -> gain_c_out/1
  ChannelOut/3 -> gain_real_out/1
  ChannelIn/1 -> ChannelOut/1
  ChannelIn/2 -> ChannelOut/2
  Mult/1 -> ChannelOut/3
  Mult1/1 -> ChannelOut/4
  ChannelOut/4 -> gain_img_out/1

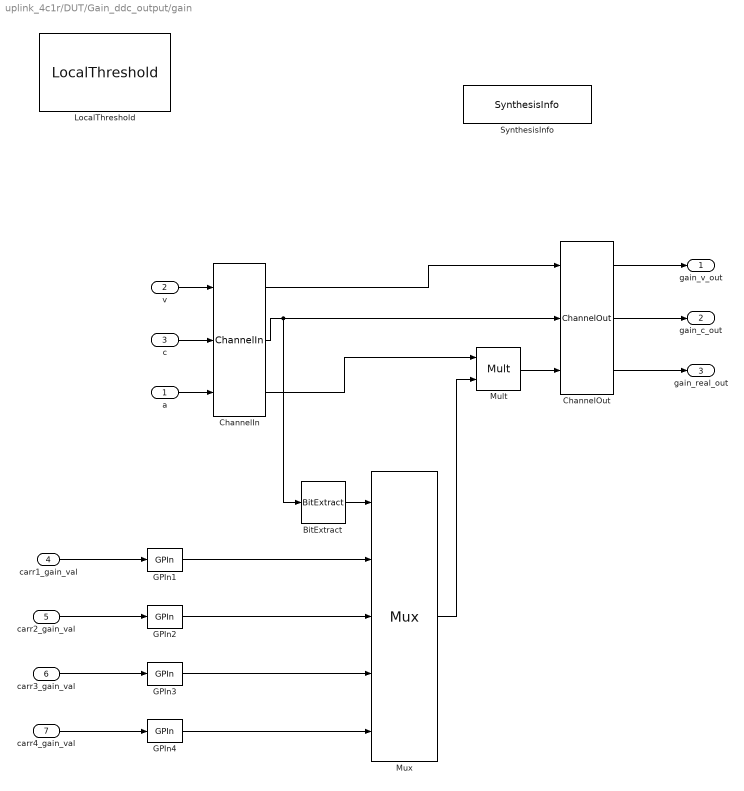
== system uplink_4c1r/DUT/Gain_ddc_output/gain ==
  a : Inport
  v : Inport  Port=2
  c : Inport  Port=3
  carr1_gain_val : Inport  Port=4
  carr2_gain_val : Inport  Port=5
  carr3_gain_val : Inport  Port=6
  carr4_gain_val : Inport  Port=7
  BitExtract : DSPBAPrim/BitExtract  primtype=bitextract  nInputs=1  nOutputs=1  omode=Specify via dialog  otype=ufix(3)  scale=2^-0  rndmethod=Unbiased  factor=1  satmethod=Symmetric  shift_vec=[0 1 2 -1]  value=1  inPortNames=[' '; ' ';]  outPortNames=[' ']  dspbaimage=dspba_prim.jpg  text=fprintf('..%d', value);  style=Optimised  visibilities=8+1024  version=20090407
  ChannelIn : DSPBAPrim/ChannelIn  primtype=channelin  nInputs=dspba_internal_get_channel_ports(gcb)  nOutputs=dspba_internal_get_channel_ports(gcb)  omode=Inherit via internal rule  otype=sfix(16)  scale=2^-15  rndmethod=Unbiased  factor=1  satmethod=Symmetric  shift_vec=[0 1 2 -1]  value=1  inPortNames=['v'; 'c'; '0'; '1'; '2'; '3'; '4'; '5'; '6'; '7'; '8'; '9'; 'A'; 'B'; 'D'; 'E'; 'F'; 'G'; 'H'; 'I'; 'J'; 'K'; 'L'; 'M'; 'N'; 'O'; 'P'; 'Q'; 'R'; 'S'; 'T'; 'U'; 'W'; 'X'; 'Y'; 'Z']  outPortNames=['v'; 'c'; '0'; '1'; '2'; '3'; '4'; '5'; '6'; '7'; '8'; '9'; 'A'; 'B'; 'D'; 'E'; 'F'; 'G'; 'H'; 'I'; 'J'; 'K'; 'L'; 'M'; 'N'; 'O'; 'P'; 'Q'; 'R'; 'S'; 'T'; 'U'; 'W'; 'X'; 'Y'; 'Z']  dspbaimage=dspba_prim.jpg  text=fprintf('In');  style=Optimised  dataSignals=1  foldingEnabled=off  channels=1  sampleRate=200  packetBeginPresent=off  packetBeginEnabled=off  visibilities=dspba_ChannelInVis(gcb)  latencyCorrection=0  version=20141013
  ChannelOut : DSPBAPrim/ChannelOut  primtype=channelout  nInputs=dspba_internal_get_channel_ports(gcb)  nOutputs=dspba_internal_get_channel_ports(gcb)  omode=Inherit via internal rule  otype=sfix(16)  scale=2^-15  rndmethod=Unbiased  factor=1  satmethod=Symmetric  shift_vec=[0 1 2 -1]  value=1  inPortNames=['v'; 'c'; '0'; '1'; '2'; '3'; '4'; '5'; '6'; '7'; '8'; '9'; 'A'; 'B'; 'D'; 'E'; 'F'; 'G'; 'H'; 'I'; 'J'; 'K'; 'L'; 'M'; 'N'; 'O'; 'P'; 'Q'; 'R'; 'S'; 'T'; 'U'; 'W'; 'X'; 'Y'; 'Z']  outPortNames=['v'; 'c'; '0'; '1'; '2'; '3'; '4'; '5'; '6'; '7'; '8'; '9'; 'A'; 'B'; 'D'; 'E'; 'F'; 'G'; 'H'; 'I'; 'J'; 'K'; 'L'; 'M'; 'N'; 'O'; 'P'; 'Q'; 'R'; 'S'; 'T'; 'U'; 'W'; 'X'; 'Y'; 'Z']  dspbaimage=dspba_prim.jpg  text=fprintf('Out%s', AdvDSPBChannelOutDisplay(latency));  style=Optimised  dataSignals=1  foldingEnabled=off  channels=1  sampleRate=200  packetBeginPresent=off  packetBeginEnabled=off  visibilities=dspba_ChannelOutVis(gcb)  latency=21  latencyCorrection=0  version=20141013
  GPIn{1..4} (4 alike) : DSPBAPrim/GPIn  primtype=gpin  nInputs=evalAionMaskParam(gcb,'value',1)  nOutputs=evalAionMaskParam(gcb,'value',1)  omode=Inherit via internal rule  otype=sfix(16)  scale=2^-15  rndmethod=Unbiased  factor=1  satmethod=Symmetric  shift_vec=[0 1 2 -1]  value=1  inPortNames=[' ' ' ' ' ' ' ' ' ' ' ' ' ' ' ' ' ' ' ' ' ' ' ' ' ' ' ' ' ' ' ' ' ' ' ' ' ' ' ' ' ' ' ' ' ' ' ' ' ' ' ' ' ' ' ' ' ' ' ' ' ' ' ' ' ' ' ' ' ']'  outPortNames=[' ' ' ' ' ' ' ' ' ' ' ' ' ' ' ' ' ' ' ' ' ' ' ' ' ' ' ' ' ' ' ' ' ' ' ' ' ' ' ' ' ' ' ' ' ' ' ' ' ' ' ' ' ' ' ' ' ' ' ' ' ' ' ' ' ' ' ' ' ']'  dspbaimage=dspba_prim.jpg  text=fprintf('GPIn');  style=Optimised  visibilities=1024  latencyCorrection=0  version=20090407
  LocalThreshold : DSPBABase/LocalThreshold  margin=DDC_Lineup_param.ClockMargin  delayRegOrRAMThresholdBits=-1  MediumDualMemThresholdBits=-1  LargeDualMemThresholdBits=-1  hardMultiplierThresholdLuts=-1  complexMultKaratsuba=off  version=0
  Mult : DSPBAPrim/Mult  primtype=mult  nInputs=2  nOutputs=1  omode=Inherit via internal rule  otype=sfix(16)  scale=2^-15  rndmethod=Unbiased  factor=1  satmethod=Symmetric  shift_vec=[0 1 2 -1]  value=0  inPortNames=[' '; ' ';]  outPortNames=[' ']  dspbaimage=dspba_prim.jpg  text=fprintf('X');  style=Optimised  visibilities=8+2^18+2^19  floatPrecision=float32_m23  floatRounding=correct  advOptions=[]  version=20130115
  Mux : DSPBAPrim/Mux  primtype=mux  nInputs=evalAionMaskParam(gcb,'value',1)+1  nOutputs=1  omode=Inherit via internal rule  otype=sfix(16)  scale=2^-15  rndmethod=Unbiased  factor=1  satmethod=Symmetric  shift_vec=[0 1 2 -1]  value=4  inPortNames=['s '; 'd0'; 'd1'; 'd2'; 'd3'; 'd4'; 'd5'; 'd6'; 'd7'; 'd8'; 'd9';]  outPortNames=[' ']  dspbaimage=dspba_prim.jpg  text=fprintf('%s', primtype);  style=Optimised  visibilities=1032  version=20131025
  SynthesisInfo : DSPBAPrim/SynthesisInfo  primtype=synthinfo  nInputs=0  nOutputs=0  omode=Inherit via internal rule  otype=sfix(16)  scale=2^-15  rndmethod=Truncate  factor=1  satmethod=Symmetric  shift_vec=[0 1 2 -1]  value=99  inPortNames=[' '; ' ';]  outPortNames=[' ']  dspbaimage=dspba_prim_ctrl.jpg  text=fprintf('Style=%s', style);  style=Scheduled  visibilities=2^15+2^17+2^18+2^19  constraintInUse=on  constraintRelation=>  constraintLimit=20  bitAccurate=off  version=20150220
  gain_v_out : Outport
  gain_c_out : Outport  Port=2
  gain_real_out : Outport  Port=3
  wires:
  carr3_gain_val/1 -> GPIn3/1
  BitExtract/1 -> Mux/1
  Mult/1 -> ChannelOut/3
  ChannelIn/2 -> ChannelOut/2, BitExtract/1
  ChannelIn/1 -> ChannelOut/1
  a/1 -> ChannelIn/3
  c/1 -> ChannelIn/2
  v/1 -> ChannelIn/1
  Mux/1 -> Mult/2
  ChannelOut/3 -> gain_real_out/1
  carr1_gain_val/1 -> GPIn1/1
  carr4_gain_val/1 -> GPIn4/1
  carr2_gain_val/1 -> GPIn2/1
  ChannelIn/3 -> Mult/1
  ChannelOut/1 -> gain_v_out/1
  ChannelOut/2 -> gain_c_out/1
  GPIn1/1 -> Mux/2
  GPIn2/1 -> Mux/3
  GPIn3/1 -> Mux/4
  GPIn4/1 -> Mux/5

== system uplink_4c1r/DUT/Power_Meter_ddc_in/carrier_separation ==
  valid : Inport
  channel : Inport  Port=2
  "data " : Inport  Port=3
  "1ms_pulse_in " : Inport  Port=4
  Add : DSPBAPrim/Add  primtype=add  nInputs=evalAionMaskParam(gcb,'value',1)  nOutputs=1  omode=Inherit via internal rule with word growth  otype=sfix(16)  scale=2^-15  rndmethod=Unbiased  factor=1  satmethod=Symmetric  shift_vec=[0 1 2 -1]  value=2  inPortNames=[' '; ' ';]  outPortNames=[' ']  dspbaimage=dspba_prim.jpg  text=fprintf('+');  style=Optimised  visibilities=1032+2^17+2^18+2^19  genFPC=off  floatRounding=correct  advOptions=[]  version=20130821
  ChannelIn : DSPBAPrim/ChannelIn  primtype=channelin  nInputs=dspba_internal_get_channel_ports(gcb)  nOutputs=dspba_internal_get_channel_ports(gcb)  omode=Inherit via internal rule  otype=sfix(16)  scale=2^-15  rndmethod=Unbiased  factor=1  satmethod=Symmetric  shift_vec=[0 1 2 -1]  value=2  inPortNames=['v'; 'c'; '0'; '1'; '2'; '3'; '4'; '5'; '6'; '7'; '8'; '9'; 'A'; 'B'; 'D'; 'E'; 'F'; 'G'; 'H'; 'I'; 'J'; 'K'; 'L'; 'M'; 'N'; 'O'; 'P'; 'Q'; 'R'; 'S'; 'T'; 'U'; 'W'; 'X'; 'Y'; 'Z']  outPortNames=['v'; 'c'; '0'; '1'; '2'; '3'; '4'; '5'; '6'; '7'; '8'; '9'; 'A'; 'B'; 'D'; 'E'; 'F'; 'G'; 'H'; 'I'; 'J'; 'K'; 'L'; 'M'; 'N'; 'O'; 'P'; 'Q'; 'R'; 'S'; 'T'; 'U'; 'W'; 'X'; 'Y'; 'Z']  dspbaimage=dspba_prim.jpg  text=fprintf('In');  style=Optimised  dataSignals=2  foldingEnabled=off  channels=1  sampleRate=200  packetBeginPresent=off  packetBeginEnabled=off  visibilities=dspba_ChannelInVis(gcb)  latencyCorrection=0  version=20141013
  ChannelOut : DSPBAPrim/ChannelOut  primtype=channelout  nInputs=dspba_internal_get_channel_ports(gcb)  nOutputs=dspba_internal_get_channel_ports(gcb)  omode=Inherit via internal rule  otype=sfix(16)  scale=2^-15  rndmethod=Unbiased  factor=1  satmethod=Symmetric  shift_vec=[0 1 2 -1]  value=2  inPortNames=['v'; 'c'; '0'; '1'; '2'; '3'; '4'; '5'; '6'; '7'; '8'; '9'; 'A'; 'B'; 'D'; 'E'; 'F'; 'G'; 'H'; 'I'; 'J'; 'K'; 'L'; 'M'; 'N'; 'O'; 'P'; 'Q'; 'R'; 'S'; 'T'; 'U'; 'W'; 'X'; 'Y'; 'Z']  outPortNames=['v'; 'c'; '0'; '1'; '2'; '3'; '4'; '5'; '6'; '7'; '8'; '9'; 'A'; 'B'; 'D'; 'E'; 'F'; 'G'; 'H'; 'I'; 'J'; 'K'; 'L'; 'M'; 'N'; 'O'; 'P'; 'Q'; 'R'; 'S'; 'T'; 'U'; 'W'; 'X'; 'Y'; 'Z']  dspbaimage=dspba_prim.jpg  text=fprintf('Out%s', AdvDSPBChannelOutDisplay(latency));  style=Optimised  dataSignals=2  foldingEnabled=off  channels=1  sampleRate=200  packetBeginPresent=off  packetBeginEnabled=off  visibilities=dspba_ChannelOutVis(gcb)  latency=21  latencyCorrection=0  version=20141013
  Demux : Demux  Outputs=2
  Mult : DSPBAPrim/Mult  primtype=mult  nInputs=2  nOutputs=1  omode=Inherit via internal rule  otype=sfix(16)  scale=2^-15  rndmethod=Unbiased  factor=1  satmethod=Symmetric  shift_vec=[0 1 2 -1]  value=0  inPortNames=[' '; ' ';]  outPortNames=[' ']  dspbaimage=dspba_prim.jpg  text=fprintf('X');  style=Optimised  visibilities=8+2^18+2^19  floatPrecision=float32_m23  floatRounding=correct  advOptions=[]  version=20130115
  Mult1 : DSPBAPrim/Mult  primtype=mult  nInputs=2  nOutputs=1  omode=Inherit via internal rule  otype=sfix(16)  scale=2^-15  rndmethod=Unbiased  factor=1  satmethod=Symmetric  shift_vec=[0 1 2 -1]  value=0  inPortNames=[' '; ' ';]  outPortNames=[' ']  dspbaimage=dspba_prim.jpg  text=fprintf('X');  style=Optimised  visibilities=8+2^18+2^19  floatPrecision=float32_m23  floatRounding=correct  advOptions=[]  version=20130115
  SynthesisInfo : DSPBAPrim/SynthesisInfo  primtype=synthinfo  nInputs=0  nOutputs=0  omode=Inherit via internal rule  otype=sfix(16)  scale=2^-15  rndmethod=Truncate  factor=1  satmethod=Symmetric  shift_vec=[0 1 2 -1]  value=99  inPortNames=[' '; ' ';]  outPortNames=[' ']  dspbaimage=dspba_prim_ctrl.jpg  text=fprintf('Style=%s', style);  style=Scheduled  visibilities=32768  constraintInUse=on  constraintRelation=>  constraintLimit=Latency  bitAccurate=off  version=20150220
  latch_0L : DSPBAControl/latch_0L
  "axc1_data_out " : Outport
  valid_out : Outport  Port=2
  channel_out : Outport  Port=3
  pulse_1ms_out : Outport  Port=4
  wires:
  Demux/2 -> Mult1/2, Mult1/1
  Demux/1 -> Mult/1, Mult/2
  ChannelIn/3 -> Demux/1
  ChannelOut/4 -> pulse_1ms_out/1
  ChannelOut/1 -> valid_out/1
  ChannelOut/2 -> channel_out/1
  ChannelOut/3 -> "axc1_data_out "/1
  ChannelIn/2 -> ChannelOut/2
  latch_0L/1 -> ChannelOut/3
  Add/1 -> latch_0L/2
  Mult1/1 -> Add/2
  Mult/1 -> Add/1
  ChannelIn/4 -> ChannelOut/4
  "data "/1 -> ChannelIn/3
  valid/1 -> ChannelIn/1
  channel/1 -> ChannelIn/2
  ChannelIn/1 -> ChannelOut/1, latch_0L/1
  "1ms_pulse_in "/1 -> ChannelIn/4

== system uplink_4c1r/DUT/Power_Meter_ddc_out/Carrier1 ==
  a : Inport
  v : Inport  Port=2
  c : Inport  Port=3
  Pulse_In : Inport  Port=4
  Reg_Busy_Bit : Inport  Port=5
  Const : DSPBAPrim/Const  primtype=const  nInputs=0  nOutputs=1  omode=Inherit via internal rule  otype=sfix(16)  scale=2^-15  rndmethod=Unbiased  factor=1  satmethod=Symmetric  shift_vec=[0 1 2 -1]  value=0  inPortNames=['+'; '+';]  outPortNames=[' ']  dspbaimage=dspba_prim.jpg  text=fprintf('%s', num2str(value));  style=Optimised  visibilities=8 + 1024  floatPrecision=float32_m23  version=20120820
  Reg_Block : uplink_4c1r_register/Reg_Block  Peak_Detector_address=0  Accumulator1_addr=1  Accumulator2_addr=2
  Scale : DSPBABase/Scale  otype=sfix(16)  scale=2^-15  rndmethod=Unbiased  factor=1  satmethod=Symmetric  shift_vec=0  latency=6  wideSimulation=off  version=20130807
  Terminator1 : Terminator
  accumulator : uplink_4c1r_accumulator/accumulator  Latency=0
      link override ChannelOut: latency=4
  peak_detector : uplink_4c1r_peak_detector/peak_detector  Latency=0
      link override ChannelOut: latency=1
  wires:
  peak_detector/2 -> Reg_Block/3
  Pulse_In/1 -> accumulator/4, peak_detector/4
  Reg_Busy_Bit/1 -> Reg_Block/4
  c/1 -> Scale/3
  Scale/2 -> accumulator/2, peak_detector/2
  Scale/4 -> Terminator1/1
  v/1 -> Scale/2
  accumulator/1 -> Reg_Block/2
  a/1 -> Scale/1
  peak_detector/1 -> Reg_Block/1
  Scale/1 -> accumulator/1, peak_detector/1
  Const/1 -> Scale/4
  Scale/3 -> accumulator/3, peak_detector/3

== system uplink_4c1r/DUT/Power_Meter_ddc_out/Carrier2 ==
  a : Inport
  v : Inport  Port=2
  c : Inport  Port=3
  Pulse_In : Inport  Port=4
  Reg_Busy_Bit : Inport  Port=5
  Const : DSPBAPrim/Const  primtype=const  nInputs=0  nOutputs=1  omode=Inherit via internal rule  otype=sfix(16)  scale=2^-15  rndmethod=Unbiased  factor=1  satmethod=Symmetric  shift_vec=[0 1 2 -1]  value=0  inPortNames=['+'; '+';]  outPortNames=[' ']  dspbaimage=dspba_prim.jpg  text=fprintf('%s', num2str(value));  style=Optimised  visibilities=8 + 1024  floatPrecision=float32_m23  version=20120820
  Reg_Block : uplink_4c1r_register/Reg_Block  Peak_Detector_address=3  Accumulator1_addr=4  Accumulator2_addr=5
  Scale : DSPBABase/Scale  otype=sfix(16)  scale=2^-15  rndmethod=Unbiased  factor=1  satmethod=Symmetric  shift_vec=0  latency=6  wideSimulation=off  version=20130807
  Terminator1 : Terminator
  accumulator : uplink_4c1r_accumulator/accumulator  Latency=0
      link override ChannelOut: latency=4
  peak_detector : uplink_4c1r_peak_detector/peak_detector  Latency=0
      link override ChannelOut: latency=1
  wires:
  peak_detector/2 -> Reg_Block/3
  Pulse_In/1 -> accumulator/4, peak_detector/4
  Reg_Busy_Bit/1 -> Reg_Block/4
  c/1 -> Scale/3
  Scale/2 -> accumulator/2, peak_detector/2
  Scale/4 -> Terminator1/1
  v/1 -> Scale/2
  accumulator/1 -> Reg_Block/2
  a/1 -> Scale/1
  peak_detector/1 -> Reg_Block/1
  Scale/1 -> accumulator/1, peak_detector/1
  Const/1 -> Scale/4
  Scale/3 -> accumulator/3, peak_detector/3

== system uplink_4c1r/DUT/Power_Meter_ddc_out/Carrier3 ==
  a : Inport
  v : Inport  Port=2
  c : Inport  Port=3
  Pulse_In : Inport  Port=4
  Reg_Busy_Bit : Inport  Port=5
  Const : DSPBAPrim/Const  primtype=const  nInputs=0  nOutputs=1  omode=Inherit via internal rule  otype=sfix(16)  scale=2^-15  rndmethod=Unbiased  factor=1  satmethod=Symmetric  shift_vec=[0 1 2 -1]  value=0  inPortNames=['+'; '+';]  outPortNames=[' ']  dspbaimage=dspba_prim.jpg  text=fprintf('%s', num2str(value));  style=Optimised  visibilities=8 + 1024  floatPrecision=float32_m23  version=20120820
  Reg_Block : uplink_4c1r_register/Reg_Block  Peak_Detector_address=6  Accumulator1_addr=7  Accumulator2_addr=8
  Scale : DSPBABase/Scale  otype=sfix(16)  scale=2^-15  rndmethod=Unbiased  factor=1  satmethod=Symmetric  shift_vec=0  latency=6  wideSimulation=off  version=20130807
  Terminator1 : Terminator
  accumulator : uplink_4c1r_accumulator/accumulator  Latency=0
      link override ChannelOut: latency=4
  peak_detector : uplink_4c1r_peak_detector/peak_detector  Latency=0
      link override ChannelOut: latency=1
  wires:
  peak_detector/2 -> Reg_Block/3
  Pulse_In/1 -> accumulator/4, peak_detector/4
  Reg_Busy_Bit/1 -> Reg_Block/4
  c/1 -> Scale/3
  Scale/2 -> accumulator/2, peak_detector/2
  Scale/4 -> Terminator1/1
  v/1 -> Scale/2
  accumulator/1 -> Reg_Block/2
  a/1 -> Scale/1
  peak_detector/1 -> Reg_Block/1
  Scale/1 -> accumulator/1, peak_detector/1
  Const/1 -> Scale/4
  Scale/3 -> accumulator/3, peak_detector/3

== system uplink_4c1r/DUT/Power_Meter_ddc_out/Carrier4 ==
  a : Inport
  v : Inport  Port=2
  c : Inport  Port=3
  Pulse_In : Inport  Port=4
  Reg_Busy_Bit : Inport  Port=5
  Const : DSPBAPrim/Const  primtype=const  nInputs=0  nOutputs=1  omode=Inherit via internal rule  otype=sfix(16)  scale=2^-15  rndmethod=Unbiased  factor=1  satmethod=Symmetric  shift_vec=[0 1 2 -1]  value=0  inPortNames=['+'; '+';]  outPortNames=[' ']  dspbaimage=dspba_prim.jpg  text=fprintf('%s', num2str(value));  style=Optimised  visibilities=8 + 1024  floatPrecision=float32_m23  version=20120820
  Reg_Block : uplink_4c1r_register/Reg_Block  Peak_Detector_address=9  Accumulator1_addr=10  Accumulator2_addr=11
  Scale : DSPBABase/Scale  otype=sfix(16)  scale=2^-15  rndmethod=Unbiased  factor=1  satmethod=Symmetric  shift_vec=0  latency=6  wideSimulation=off  version=20130807
  Terminator1 : Terminator
  accumulator : uplink_4c1r_accumulator/accumulator  Latency=0
      link override ChannelOut: latency=4
  peak_detector : uplink_4c1r_peak_detector/peak_detector  Latency=0
      link override ChannelOut: latency=1
  wires:
  peak_detector/2 -> Reg_Block/3
  Pulse_In/1 -> accumulator/4, peak_detector/4
  Reg_Busy_Bit/1 -> Reg_Block/4
  c/1 -> Scale/3
  Scale/2 -> accumulator/2, peak_detector/2
  Scale/4 -> Terminator1/1
  v/1 -> Scale/2
  accumulator/1 -> Reg_Block/2
  a/1 -> Scale/1
  peak_detector/1 -> Reg_Block/1
  Scale/1 -> accumulator/1, peak_detector/1
  Const/1 -> Scale/4
  Scale/3 -> accumulator/3, peak_detector/3

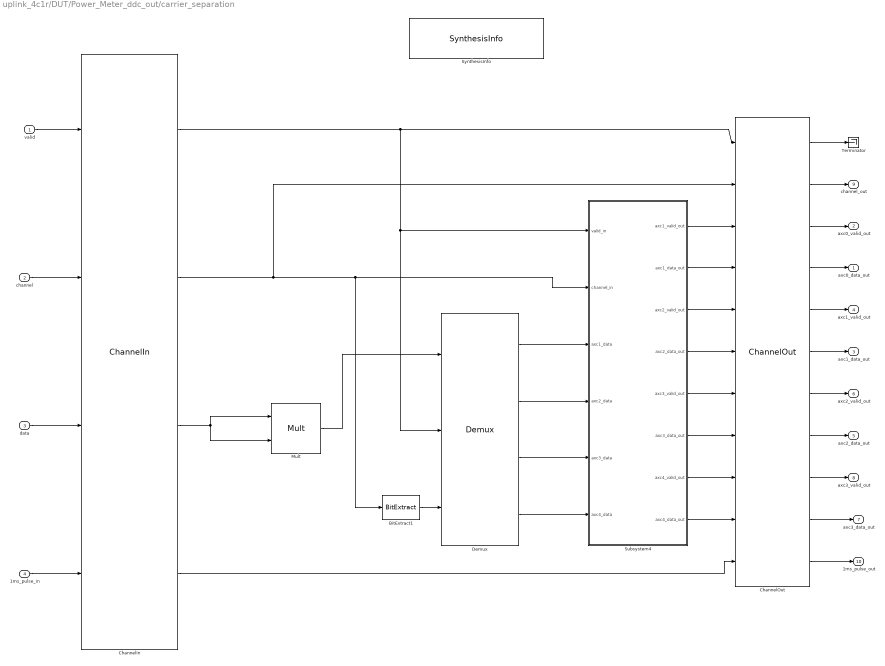
== system uplink_4c1r/DUT/Power_Meter_ddc_out/carrier_separation ==
  valid : Inport
  channel : Inport  Port=2
  "data " : Inport  Port=3
  "1ms_pulse_in " : Inport  Port=4
  BitExtract1 : DSPBAPrim/BitExtract  primtype=bitextract  nInputs=1  nOutputs=1  omode=Specify via dialog  otype=ufix(4)  scale=2^0  rndmethod=Unbiased  factor=1  satmethod=Symmetric  shift_vec=[0 1 2 -1]  value=1  inPortNames=[' '; ' ';]  outPortNames=[' ']  dspbaimage=dspba_prim.jpg  text=fprintf('..%d', value);  style=Optimised  visibilities=8 + 1024  version=20090407
  ChannelIn : DSPBAPrim/ChannelIn  primtype=channelin  nInputs=dspba_internal_get_channel_ports(gcb)  nOutputs=dspba_internal_get_channel_ports(gcb)  omode=Inherit via internal rule  otype=sfix(16)  scale=2^-15  rndmethod=Unbiased  factor=1  satmethod=Symmetric  shift_vec=[0 1 2 -1]  value=2  inPortNames=['v'; 'c'; '0'; '1'; '2'; '3'; '4'; '5'; '6'; '7'; '8'; '9'; 'A'; 'B'; 'D'; 'E'; 'F'; 'G'; 'H'; 'I'; 'J'; 'K'; 'L'; 'M'; 'N'; 'O'; 'P'; 'Q'; 'R'; 'S'; 'T'; 'U'; 'W'; 'X'; 'Y'; 'Z']  outPortNames=['v'; 'c'; '0'; '1'; '2'; '3'; '4'; '5'; '6'; '7'; '8'; '9'; 'A'; 'B'; 'D'; 'E'; 'F'; 'G'; 'H'; 'I'; 'J'; 'K'; 'L'; 'M'; 'N'; 'O'; 'P'; 'Q'; 'R'; 'S'; 'T'; 'U'; 'W'; 'X'; 'Y'; 'Z']  dspbaimage=dspba_prim.jpg  text=fprintf('In');  style=Optimised  dataSignals=2  foldingEnabled=off  channels=1  sampleRate=200  packetBeginPresent=off  packetBeginEnabled=off  visibilities=dspba_ChannelInVis(gcb)  latencyCorrection=0  version=20141013
  ChannelOut : DSPBAPrim/ChannelOut  primtype=channelout  nInputs=dspba_internal_get_channel_ports(gcb)  nOutputs=dspba_internal_get_channel_ports(gcb)  omode=Inherit via internal rule  otype=sfix(16)  scale=2^-15  rndmethod=Unbiased  factor=1  satmethod=Symmetric  shift_vec=[0 1 2 -1]  value=9  inPortNames=['v'; 'c'; '0'; '1'; '2'; '3'; '4'; '5'; '6'; '7'; '8'; '9'; 'A'; 'B'; 'D'; 'E'; 'F'; 'G'; 'H'; 'I'; 'J'; 'K'; 'L'; 'M'; 'N'; 'O'; 'P'; 'Q'; 'R'; 'S'; 'T'; 'U'; 'W'; 'X'; 'Y'; 'Z']  outPortNames=['v'; 'c'; '0'; '1'; '2'; '3'; '4'; '5'; '6'; '7'; '8'; '9'; 'A'; 'B'; 'D'; 'E'; 'F'; 'G'; 'H'; 'I'; 'J'; 'K'; 'L'; 'M'; 'N'; 'O'; 'P'; 'Q'; 'R'; 'S'; 'T'; 'U'; 'W'; 'X'; 'Y'; 'Z']  dspbaimage=dspba_prim.jpg  text=fprintf('Out%s', AdvDSPBChannelOutDisplay(latency));  style=Optimised  dataSignals=9  foldingEnabled=off  channels=1  sampleRate=200  packetBeginPresent=off  packetBeginEnabled=off  visibilities=dspba_ChannelOutVis(gcb)  latency=21  latencyCorrection=0  version=20141013
  Demux : DSPBAPrim/Demux  primtype=demux  nInputs=3  nOutputs=dspba_internal_get_demux_ports(gcb)  omode=Inherit via internal rule  otype=sfix(16)  scale=2^-15  rndmethod=Unbiased  factor=1  satmethod=Symmetric  shift_vec=[0 1 2 3]  value=4  inPortNames=['q'; 'v'; 'c']  outPortNames=['c0'; 'c1']  dspbaimage=dspba_prim.jpg  text=fprintf('demux');  style=Optimised  visibilities=1536  version=20100120
  Mult : DSPBAPrim/Mult  primtype=mult  nInputs=2  nOutputs=1  omode=Inherit via internal rule  otype=sfix(16)  scale=2^-15  rndmethod=Unbiased  factor=1  satmethod=Symmetric  shift_vec=[0 1 2 -1]  value=0  inPortNames=[' '; ' ';]  outPortNames=[' ']  dspbaimage=dspba_prim.jpg  text=fprintf('X');  style=Optimised  visibilities=8+2^18+2^19  floatPrecision=float32_m23  floatRounding=correct  advOptions=[]  version=20130115
  Subsystem4 : Subsystem
  SynthesisInfo : DSPBAPrim/SynthesisInfo  primtype=synthinfo  nInputs=0  nOutputs=0  omode=Inherit via internal rule  otype=sfix(16)  scale=2^-15  rndmethod=Truncate  factor=1  satmethod=Symmetric  shift_vec=[0 1 2 -1]  value=99  inPortNames=[' '; ' ';]  outPortNames=[' ']  dspbaimage=dspba_prim_ctrl.jpg  text=fprintf('Style=%s', style);  style=Scheduled  visibilities=32768  constraintInUse=on  constraintRelation=>  constraintLimit=Latency  bitAccurate=off  version=20150220
  Terminator : Terminator
  "axc0_data_out " : Outport
  axc0_valid_out : Outport  Port=2
  axc1_data_out : Outport  Port=3
  axc1_valid_out : Outport  Port=4
  axc2_data_out : Outport  Port=5
  axc2_valid_out : Outport  Port=6
  axc3_data_out : Outport  Port=7
  axc3_valid_out : Outport  Port=8
  channel_out : Outport  Port=9
  1ms_pulse_out : Outport  Port=10
  wires:
  Subsystem4/8(axc4_data_out) -> ChannelOut/10
  Subsystem4/7(axc4_valid_out) -> ChannelOut/9
  Subsystem4/6(axc3_data_out) -> ChannelOut/8
  Subsystem4/5(axc3_valid_out) -> ChannelOut/7
  Subsystem4/4(axc2_data_out) -> ChannelOut/6
  Subsystem4/3(axc2_valid_out) -> ChannelOut/5
  Subsystem4/2("axc1_data_out ") -> ChannelOut/4
  Subsystem4/1(axc1_valid_out) -> ChannelOut/3
  Demux/4 -> Subsystem4/6(axc4_data)
  Demux/3 -> Subsystem4/5(axc3_data)
  Demux/2 -> Subsystem4/4(axc2_data)
  Demux/1 -> Subsystem4/3(axc1_data)
  ChannelIn/3 -> Mult/2, Mult/1
  ChannelOut/2 -> channel_out/1
  "data "/1 -> ChannelIn/3
  ChannelOut/1 -> Terminator/1
  valid/1 -> ChannelIn/1
  channel/1 -> ChannelIn/2
  BitExtract1/1 -> Demux/3
  Mult/1 -> Demux/1
  ChannelIn/1 -> ChannelOut/1, Subsystem4/1(valid_in), Demux/2
  ChannelIn/2 -> ChannelOut/2, BitExtract1/1, Subsystem4/2(channel_in)
  ChannelOut/4 -> "axc0_data_out "/1
  ChannelOut/9 -> axc3_valid_out/1
  ChannelOut/3 -> axc0_valid_out/1
  ChannelOut/5 -> axc1_valid_out/1
  ChannelOut/6 -> axc1_data_out/1
  ChannelOut/7 -> axc2_valid_out/1
  ChannelOut/8 -> axc2_data_out/1
  ChannelOut/10 -> axc3_data_out/1
  ChannelIn/4 -> ChannelOut/11
  ChannelOut/11 -> 1ms_pulse_out/1
  "1ms_pulse_in "/1 -> ChannelIn/4
